simulink model "Introduction_simulink"  (R2018a)
settings: Solver=VariableStepAuto  StartTime=0.0  StopTime=300  RelTol=1e-3
values from neighbouring files (symbols this model uses):
  g = 9.8    [Introduction_simulink_para.m]
  k = 0.01    [DC_motor_speed_para.m]    (also in Introduction_simulink_para.m = 1)
  m1 = 1    [Introduction_simulink_para.m]
  m2 = 0.5    [Introduction_simulink_para.m]
  mu = 0.02    [Introduction_simulink_para.m]
undefined symbols (not defined in the file or in its folder): sigbuilder_block
libraries: simulink x1
settings Model: Creator=Infi  LastModifiedBy=Infi

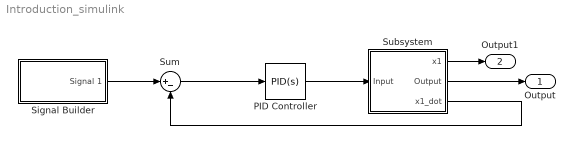
== system Introduction_simulink ==
  PID Controller : simulink/Continuous/PID Controller  Controller=PID  TimeDomain=Continuous-time  SampleTime=-1  IntegratorMethod=Forward Euler  FilterMethod=Forward Euler  Form=Parallel  UseFilter=on  ControllerParametersSource=internal  P=0.266998637563713  I=0.040049795634557  D=0  N=1  InitialConditionSource=internal  InitialConditionForIntegrator=0  InitialConditionForFilter=0  ExternalReset=none  LimitOutput=off  UpperSaturationLimit=inf  LowerSaturationLimit=-inf  LinearizeAsGain=on  AntiWindupMode=none  Kb=1  TrackingMode=off  Kt=1  PParamMin=[]  PParamMax=[]  IParamMin=[]  IParamMax=[]  DParamMin=[]  DParamMax=[]  NParamMin=[]  NParamMax=[]  KbParamMin=[]  KbParamMax=[]  KtParamMin=[]  KtParamMax=[]  POutMin=[]  POutMax=[]  IOutMin=[]  IOutMax=[]  DOutMin=[]  DOutMax=[]  NOutMin=[]  NOutMax=[]  KbOutMin=[]  KbOutMax=[]  KtOutMin=[]  KtOutMax=[]  IntegratorOutMin=[]  IntegratorOutMax=[]  FilterOutMin=[]  FilterOutMax=[]  SumOutMin=[]  SumOutMax=[]  SumI1OutMin=[]  SumI1OutMax=[]  SumI2OutMin=[]  SumI2OutMax=[]  SumI3OutMin=[]  SumI3OutMax=[]  SumDOutMin=[]  SumDOutMax=[]  SaturationOutMin=[]  SaturationOutMax=[]  IntegratorContinuousStateAttributes=''  IntegratorStateMustResolveToSignalObject=off  IntegratorRTWStateStorageClass=Auto  FilterContinuousStateAttributes=''  FilterStateMustResolveToSignalObject=off  FilterRTWStateStorageClass=Auto  DifferentiatorICPrevScaledInput=0  DifferentiatorOutMin=[]  DifferentiatorOutMax=[]  FilterDiffOutCoefMin=[]  FilterDiffOutCoefMax=[]  SumDenOutMin=[]  SumDenOutMax=[]  SumNumOutMin=[]  SumNumOutMax=[]  ReciprocalOutMin=[]  ReciprocalOutMax=[]  DivideOutMin=[]  DivideOutMax=[]  TunerSelectOption=Transfer Function Based (PID Tuner App)
  Signal Builder : Subsystem  Tag=STV Subsys  LoadFcn=sigbuilder_block('load');  StartFcn=sigbuilder_block('start');  StopFcn=sigbuilder_block('stop');  ClipboardFcn=sigbuilder_block('clipboard');  mask(Sigbuilder block){tuvar=[0:10]}
      mask help: Simulink:masks:SigbuilderBlock_MD
      mask init:
      | if ~strcmp(get_param(bdroot(gcbh),'SimulationStatus'),'stopped') tuvar = sigbuilder_block('maskInit'); end
      settings: CopyFcn=sigbuilder_block('copy');  DeleteFcn=sigbuilder_block('delete');  ModelCloseFcn=sigbuilder_block('modelClose');  PreSaveFcn=sigbuilder_block('preSave');  PauseFcn=sigbuilder_block('pause');  ContinueFcn=sigbuilder_block('continue');  NameChangeFcn=sigbuilder_block('namechange');  OpenFcn=sigbuilder_block('open',[400.8 74.4 550.8 400.2 ]);  CloseFcn=sigbuilder_block('close');
      mask Display: plot(0, 0, 100, 100,[2, 2, 32, 32, 2], [68, 8, 8, 68, 68],[32, 2], [38, 38], [32, 19, 2],[53, 60, 44], [32, 17, 17, 2],[16, 16, 31, 31]);txt = getActiveGroup(gcbh);text(2, 100, txt,'verticalAlignment', 'top');
  Subsystem : Subsystem
  Sum : Sum  Inputs=|+-
  Output : Outport  SignalName=x2
  Output1 : Outport  Port=2  SignalName=x1
  wires:
  Subsystem/2(Output) -> Output/1
  PID Controller/1 -> Subsystem/1(Input)
  Subsystem/3(x1_dot) -> Sum/2
  Sum/1 -> PID Controller/1
  Signal Builder/1(Signal 1) -> Sum/1
  Subsystem/1(x1) -> Output1/1

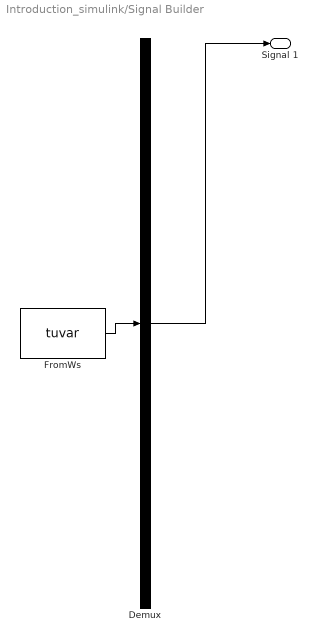
== system Introduction_simulink/Signal Builder ==
  Demux : Demux  Tag=STV Demux  Outputs=1
  FromWs : FromWorkspace  Tag=STV FromWs  VariableName=tuvar  SampleTime=0
      SigBuilderData=|
      | common.afterFinalStr = 'Extrapolate'
      | common.sampleTime = 0
      | dataSet.timeRange = [0 300]
      | dataSet.name = 'Group 1'
      | sbobj.Groups.Name = 'Group 1'
      | sbobj.Groups.Signals.Name = 'Signal 1'
      | sbobj.Groups.Signals.XData = [0 0.64 0.64 150 150 300]
      | sbobj.Groups.Signals.YData = [0 0 1 1 0 0]
      | sbobj.Groups.TimeRange = [0 300]
  Signal 1 : Outport  Tag=STV Outport
  wires:
  Demux/1 -> Signal 1/1
  FromWs/1 -> Demux/1

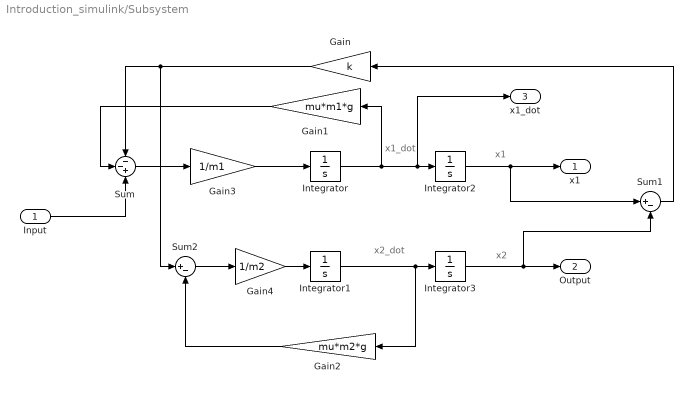
== system Introduction_simulink/Subsystem ==
  note: x2
  note: x1
  note: x2_dot
  note: x1_dot
  Input : Inport
  Gain : Gain  Gain=k
  Gain1 : Gain  Gain=mu*m1*g
  Gain2 : Gain  Gain=mu*m2*g
  Gain3 : Gain  Gain=1/m1
  Gain4 : Gain  Gain=1/m2
  Integrator{,1..3} (4 alike) : Integrator
  Sum : Sum  Inputs=--+
  Sum1 : Sum  Inputs=|+-
  Sum2 : Sum  Inputs=|+-
  x1 : Outport
  Output : Outport  Port=2
  x1_dot : Outport  Port=3
  wires:
  Gain1/1 -> Sum/2
  Integrator2/1 -> x1/1, Sum1/1
  Integrator1/1 -> Gain2/1, Integrator3/1
  Sum2/1 -> Gain4/1
  Gain/1 -> Sum2/1, Sum/1
  Integrator/1 -> Gain1/1, x1_dot/1, Integrator2/1
  Integrator3/1 -> Output/1, Sum1/2
  Gain2/1 -> Sum2/2
  Sum1/1 -> Gain/1
  Sum/1 -> Gain3/1
  Input/1 -> Sum/3
  Gain4/1 -> Integrator1/1
  Gain3/1 -> Integrator/1
